simulink model "simulierterStream_toMatlab"  (R2013b)
settings: Solver=ode45  StartTime=0.0  StopTime=10.0  RelTol=1e-3
undefined symbols (not defined in the file or in its folder): periSam, sampleTime, sigbuilder_block
libraries: simulink_extras x15, simulink x1, dspswit3 x1
settings Model: Creator=mainster  LastModifiedBy=mainster

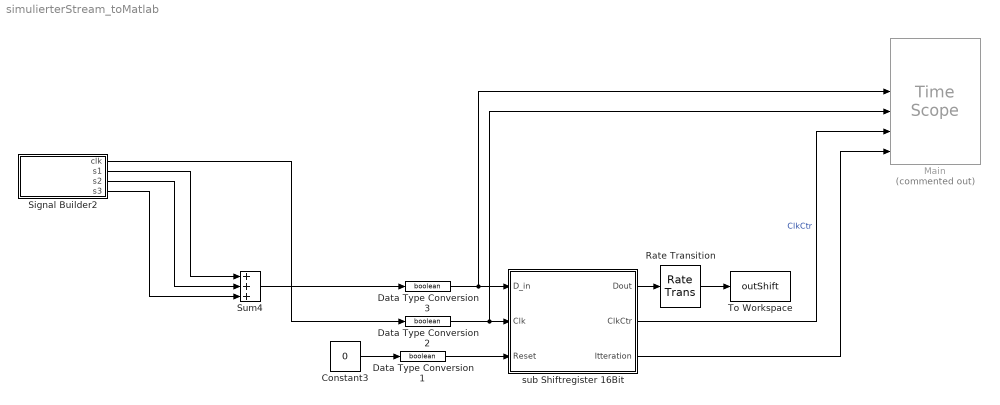
== system simulierterStream_toMatlab ==
  Constant3 : Constant  Value=0  SampleTime=-1
  Data Type Conversion1 : DataTypeConversion  OutDataTypeStr=boolean
  Data Type Conversion2 : DataTypeConversion  OutDataTypeStr=boolean
  Data Type Conversion3 : DataTypeConversion  OutDataTypeStr=boolean
  Main : TimeScope  Commented=on  NumInputPorts=6  DefaultConfigurationName=spbscopes.TimeScopeBlockCfg
      settings: CopyFcn=scopeextensions.ScopeBlock.onCoreBlockCopy(gcbh);  DeleteFcn=scopeextensions.ScopeBlock.callback(gcbh, 'onBlockDelete');  PreSaveFcn=scopeextensions.ScopeBlock.callback(gcbh, 'onModelSave');  NameChangeFcn=scopeextensions.ScopeBlock.callback(gcbh, 'onBlockRename');  DestroyFcn=scopeextensions.ScopeBlock.onBlockDestroy(gcbh)  CloseFcn=scopeextensions.ScopeBlock.callback(gcbh, 'onBlockClose');  PreDeleteFcn=scopeextensions.ScopeBlock.callback(gcbh, 'onBlockPreDelete');
  Rate Transition : RateTransition  OutPortSampleTime=sampleTime*periSam
  Signal Builder2 : Subsystem  Tag=STV Subsys  LoadFcn=sigbuilder_block('load');  StartFcn=sigbuilder_block('start');  StopFcn=sigbuilder_block('stop');  ClipboardFcn=sigbuilder_block('clipboard');  TreatAsAtomicUnit=on  mask(Sigbuilder block){}
      mask help: Simulink:masks:SigbuilderBlock_MD
      mask init:
      | if ~strcmp(get_param(bdroot(gcbh),'SimulationStatus'),'stopped') tuvar = sigbuilder_block('maskInit'); end
      settings: CopyFcn=sigbuilder_block('copy');  DeleteFcn=sigbuilder_block('delete');  ModelCloseFcn=sigbuilder_block('modelClose');  PreSaveFcn=sigbuilder_block('preSave');  PauseFcn=sigbuilder_block('pause');  ContinueFcn=sigbuilder_block('continue');  NameChangeFcn=sigbuilder_block('namechange');  OpenFcn=sigbuilder_block('open',[367.5 138 550.5 399.75 ]);  CloseFcn=sigbuilder_block('close');
      mask Display: plot(0, 0, 100, 100,[2, 2, 32, 32, 2], [68, 8, 8, 68, 68],[32, 2], [38, 38], [32, 19, 2],[53, 60, 44], [32, 17, 17, 2],[16, 16, 31, 31]);txt = getActiveGroup(gcbh);text(2, 100, txt,'verticalAlignment', 'top');
  Sum4 : Sum  Inputs=+++  SampleTime=sampleTime
  To Workspace : ToWorkspace  VariableName=outShift  SampleTime=periSam*sampleTime  SaveFormat=Timeseries
  sub Shiftregister 16Bit : Subsystem  TreatAsAtomicUnit=on
  wires:
  Signal Builder2/3(s2) -> Sum4/2
  Signal Builder2/2(s1) -> Sum4/1
  Signal Builder2/4(s3) -> Sum4/3
  Rate Transition/1 -> To Workspace/1
  Signal Builder2/1(clk) -> Data Type Conversion2/1
  Constant3/1 -> Data Type Conversion1/1
  sub Shiftregister 16Bit/1(Dout) -> Rate Transition/1
  Data Type Conversion1/1 -> sub Shiftregister 16Bit/3(Reset)
  Data Type Conversion2/1 -> Main/4, sub Shiftregister 16Bit/2(Clk)
  Data Type Conversion3/1 -> Main/3, sub Shiftregister 16Bit/1(D_in)
  Sum4/1 -> Data Type Conversion3/1
  sub Shiftregister 16Bit/3(Itteration) -> Main/6
  sub Shiftregister 16Bit/2(ClkCtr) -> Main/5  "ClkCtr"

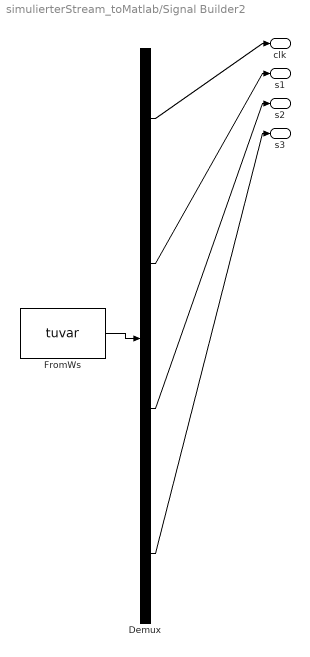
== system simulierterStream_toMatlab/Signal Builder2 ==
  Demux : Demux  Tag=STV Demux
  FromWs : FromWorkspace  Tag=STV FromWs  VariableName=tuvar  SampleTime=0
      SigBuilderData=|
      | common.afterFinalStr = 'Extrapolate'
      | common.sampleTime = 0
      | dataSet.timeRange = [0 0.00032]
      | dataSet.name = 'Group 1'
      | sbobj.Groups.Name = 'Group 1'
      | sbobj.Groups.Signals(1).Name = 'clk'
      | sbobj.Groups.Signals(1).XData = [0 1e-05 1e-05 2e-05 2e-05 3e-05 3e-05 4e-05 4e-05 5e-05 5e-05 6e-05 6e-05 7e-05 7e-05 8e-05 8e-05 9e-05 9e-05 0.0001 0.0001 0.00011 0.00011 0.00012 0.00012 0.00013 0.00013 0.00014 0.00014 0.00015 0.00015 0.00016 0.00016 0.00017 0.00017 0.00018 0.00018 0.00019 0.00019 0.0002 0.0002 0.00021 0.00021 0.00022 0.00022 0.00023 0.00023 0.00024 0.00024 0.00025 0.00025 0.00026 0.00026 0.00027 0.00027 0.00028 0.00028 0.00029 0.00029 0.0003 0.0003 0.00031 0.00031 0.00032]
      | sbobj.Groups.Signals(1).YData = [1 1 0 0 1 1 0 0 1 1 0 0 1 1 0 0 1 1 0 0 1 1 0 0 1 1 0 0 1 1 0 0 1 1 0 0 1 1 0 0 1 1 0 0 1 1 0 0 1 1 0 0 1 1 0 0 1 1 0 0 1 1 0 0]
      | sbobj.Groups.Signals(2).Name = 's1'
      | sbobj.Groups.Signals(2).XData = [0 5e-06 5e-06 5.45e-05 5.45e-05 0.00032]
      | sbobj.Groups.Signals(2).YData = [0 0 1 1 0 0]
      | sbobj.Groups.Signals(3).Name = 's2'
      | sbobj.Groups.Signals(3).XData = [0 0.0001475 0.0001475 0.000196 0.000196 0.00032]
      | sbobj.Groups.Signals(3).YData = [0 0 1 1 0 0]
      | sbobj.Groups.Signals(4).Name = 's3'
      | sbobj.Groups.Signals(4).XData = [0 0.000237 0.000237 0.000297 0.000297 0.00032]
      | sbobj.Groups.Signals(4).YData = [0 0 1 1 0 0]
      | sbobj.Groups.TimeRange = [0 0.00032]
  clk : Outport  Tag=STV Outport
  s1 : Outport  Tag=STV Outport  Port=2
  s2 : Outport  Tag=STV Outport  Port=3
  s3 : Outport  Tag=STV Outport  Port=4
  wires:
  FromWs/1 -> Demux/1
  Demux/1 -> clk/1
  Demux/2 -> s1/1
  Demux/3 -> s2/1
  Demux/4 -> s3/1

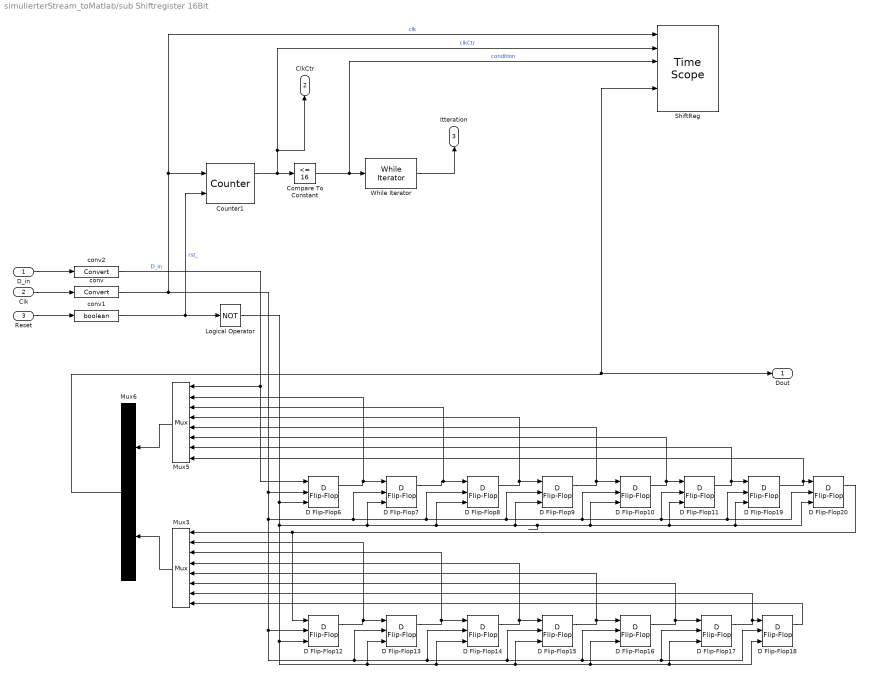
== system simulierterStream_toMatlab/sub Shiftregister 16Bit ==
  D_in : Inport
  Clk : Inport  Port=2
  Reset : Inport  Port=3
  Compare To Constant : simulink/Logic and Bit Operations/Compare To Constant  relop=<=  const=16  OutDataTypeStr=boolean  ZeroCross=off
  Counter1 : dspswit3/Counter  Direction=Up  CountEvent=Rising edge  CounterSize=User defined  MaxCount=255  InitialCount=0  Output=Count and Hit  HitValue=32  ResetInput=on  SamplesPerFrame=1  Ts=1  CntDtype=double  HitDtype=Boolean
  D Flip-Flop{6..20} (15 alike) : simulink_extras/Flip Flops/D Flip-Flop
  Logical Operator : Logic  Operator=NOT  IconShape=distinctive  AllPortsSameDT=off  OutDataTypeStr=boolean
  Mux3 : Mux  Inputs=8
  Mux5 : Mux  Inputs=8
  Mux6 : Mux  Inputs=2
  "ShiftReg " : TimeScope  NumInputPorts=6  DefaultConfigurationName=spbscopes.TimeScopeBlockCfg
      settings: CopyFcn=scopeextensions.ScopeBlock.onCoreBlockCopy(gcbh);  DeleteFcn=scopeextensions.ScopeBlock.callback(gcbh, 'onBlockDelete');  PreSaveFcn=scopeextensions.ScopeBlock.callback(gcbh, 'onModelSave');  NameChangeFcn=scopeextensions.ScopeBlock.callback(gcbh, 'onBlockRename');  DestroyFcn=scopeextensions.ScopeBlock.onBlockDestroy(gcbh)  CloseFcn=scopeextensions.ScopeBlock.callback(gcbh, 'onBlockClose');  PreDeleteFcn=scopeextensions.ScopeBlock.callback(gcbh, 'onBlockPreDelete');
  While Iterator : WhileIterator  MaxIters=1000  WhileBlockType=do-while  ResetStates=reset  ShowIterationPort=on
  conv : DataTypeConversion  LockScale=on
  conv1 : DataTypeConversion  OutDataTypeStr=boolean
  conv2 : DataTypeConversion
  Dout : Outport
  ClkCtr : Outport  Port=2
  Itteration : Outport  Port=3
  wires:
  D Flip-Flop6/1 -> Mux5/2, D Flip-Flop7/1
  D Flip-Flop7/1 -> Mux5/3, D Flip-Flop8/1
  D Flip-Flop9/1 -> Mux5/5, D Flip-Flop10/1
  D Flip-Flop10/1 -> Mux5/6, D Flip-Flop11/1
  D Flip-Flop12/1 -> Mux3/2, D Flip-Flop13/1
  D Flip-Flop13/1 -> Mux3/3, D Flip-Flop14/1
  D Flip-Flop14/1 -> Mux3/4, D Flip-Flop15/1
  D Flip-Flop17/1 -> Mux3/7, D Flip-Flop18/1
  conv/1 -> "ShiftReg "/1, Counter1/1, D Flip-Flop13/2, D Flip-Flop16/2, D Flip-Flop17/2, D Flip-Flop18/2, D Flip-Flop15/2, D Flip-Flop14/2, D Flip-Flop12/2, D Flip-Flop20/2, D Flip-Flop19/2, D Flip-Flop11/2, D Flip-Flop10/2, D Flip-Flop9/2, D Flip-Flop8/2, D Flip-Flop7/2, D Flip-Flop6/2  "clk"
  D Flip-Flop8/1 -> Mux5/4, D Flip-Flop9/1
  D Flip-Flop15/1 -> Mux3/5, D Flip-Flop16/1
  D Flip-Flop16/1 -> Mux3/6, D Flip-Flop17/1
  D Flip-Flop18/1 -> Mux3/8
  D Flip-Flop19/1 -> Mux5/8, D Flip-Flop20/1
  D Flip-Flop11/1 -> Mux5/7, D Flip-Flop19/1
  D Flip-Flop20/1 -> D Flip-Flop12/1, Mux3/1
  conv2/1 -> D Flip-Flop6/1, Mux5/1  "D_in"
  Mux5/1 -> Mux6/1
  Mux3/1 -> Mux6/2
  D_in/1 -> conv2/1
  Clk/1 -> conv/1
  Counter1/1 -> ClkCtr/1, "ShiftReg "/2, Compare To Constant/1  "clkCtr"
  Compare To Constant/1 -> While Iterator/1, "ShiftReg "/3  "condition"
  conv1/1 -> Logical Operator/1, Counter1/2  "rst_"
  Reset/1 -> conv1/1
  Logical Operator/1 -> D Flip-Flop6/3, D Flip-Flop18/3, D Flip-Flop17/3, D Flip-Flop16/3, D Flip-Flop15/3, D Flip-Flop14/3, D Flip-Flop13/3, D Flip-Flop12/3, D Flip-Flop19/3, D Flip-Flop20/3, D Flip-Flop11/3, D Flip-Flop10/3, D Flip-Flop9/3, D Flip-Flop8/3, D Flip-Flop7/3
  While Iterator/1 -> Itteration/1
  Mux6/1 -> Dout/1, "ShiftReg "/5
